simulink model "Bulker4_Main"  (R2023b)
settings: Solver=ode4  StartTime=0.0  StopTime=3600  FixedStep=0.01  RelTol=1e-3
StopFcn:
  | post_plot_bulker
undefined symbols (not defined in the file or in its folder): I, LOS, PD, S, x0, x_Curve, y_Curve
libraries: simulink x6, simulink_extras x1, mpclib x1
settings Model: SimulationMode=accelerator  Creator=HP  LastModifiedBy=myozi
settings SolverCC: AlgebraicLoopSolver=TrustRegion
settings DebuggingCC: UnconnectedInputMsg=warning  UnconnectedOutputMsg=warning  UnconnectedLineMsg=warning
settings ModelReferenceCC: EnableRefExpFcnMdlSchedulingChecks=on

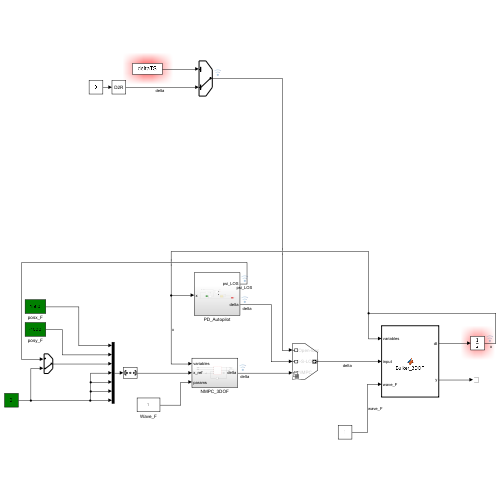
[thumbnail: Simulink's stored preview of the top-level diagram]
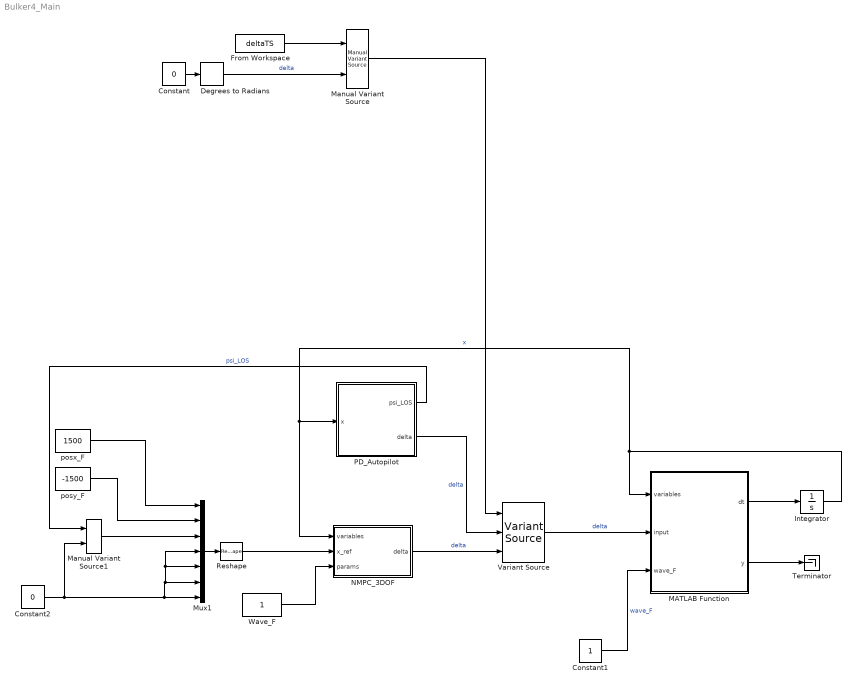
== system Bulker4_Main ==
  Constant : Constant  Value=0
  Constant1 : Constant
  Constant2 : Constant  Value=0
  Degrees to Radians : simulink_extras/Transformations/Degrees to Radians
  From Workspace : FromWorkspace  VariableName=deltaTS  OutputAfterFinalValue=Holding final value
  Integrator : Integrator  InitialCondition=x0
  MATLAB Function : MATLAB Function  TreatAsAtomicUnit=on
  Manual Variant Source : simulink/Signal Routing/Manual Variant Source  NumChoices=2  LabelModeActiveChoice=V_2
  Manual Variant Source1 : simulink/Signal Routing/Manual Variant Source  NumChoices=2  LabelModeActiveChoice=V_2
  Mux1 : Mux  Inputs=7
  NMPC_3DOF : Subsystem  VariantControl=Variant
  PD_Autopilot : Subsystem
  Reshape : Reshape  OutputDimensionality=Row vector (2-D)
  Terminator : Terminator
  Variant Source : VariantSource  VariantControlMode=label  LabelModeActiveChoice=I-S-LOS-PD  ShowConditionOnBlock=on
  Wave_F : Constant
  posx_F : Constant  Value=1500
  posy_F : Constant  Value=-1500
  wires:
  MATLAB Function/1(dt) -> Integrator/1
  Integrator/1 -> MATLAB Function/1(variables), PD_Autopilot/1(x), NMPC_3DOF/1(variables)  "x"
  Constant/1 -> Degrees to Radians/1
  Degrees to Radians/1 -> Manual Variant Source/2  "delta"
  Constant1/1 -> MATLAB Function/3(wave_F)  "wave_F"
  MATLAB Function/2(y) -> Terminator/1
  Variant Source/1 -> MATLAB Function/2(input)  "delta"
  Wave_F/1 -> NMPC_3DOF/3(params)
  Reshape/1 -> NMPC_3DOF/2(x_ref)
  NMPC_3DOF/1(delta) -> Variant Source/3  "delta"
  posy_F/1 -> Mux1/2
  Constant2/1 -> Manual Variant Source1/2, Mux1/6, Mux1/5, Mux1/4, Mux1/7
  Mux1/1 -> Reshape/1
  posx_F/1 -> Mux1/1
  PD_Autopilot/1(psi_LOS) -> Manual Variant Source1/1  "psi_LOS"
  PD_Autopilot/2(delta) -> Variant Source/2  "delta"
  Manual Variant Source1/1 -> Mux1/3
  Manual Variant Source/1 -> Variant Source/1
  From Workspace/1 -> Manual Variant Source/1

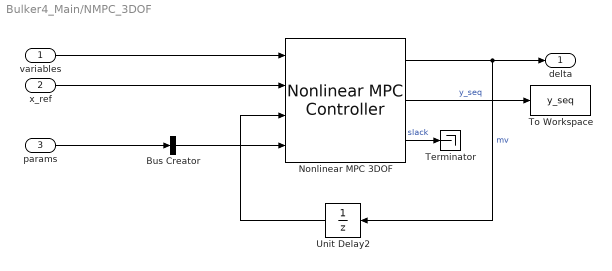
== system Bulker4_Main/NMPC_3DOF ==
  variables : Inport
  x_ref : Inport  Port=2
  params : Inport  Port=3
  Bus Creator : BusCreator  Inputs=1  OutDataTypeStr=Bus: params_bus_object  NonVirtualBus=on
      settings: InheritFromInputs=off
  Nonlinear MPC 3DOF : mpclib/Nonlinear MPC Controller  SCDEnableBlockLinearizationSpecification=on  nlmpcobj=bulker_nmpc_3_delta  UseObjectTs=off  TsControl=BlockTs  md_enabled=off  mvtarget_enabled=off  param_enabled=on  cost_enabled=off  mvseq_enabled=off  stateseq_enabled=off  ovseq_enabled=on  slack_enabled=on  status_enabled=off  ov_min=off  ov_max=off  mv_min=off  mv_max=off  mvrate_min=off  mvrate_max=off  state_min=off  state_max=off  ov_weight=off  mv_weight=off  mvrate_weight=off  ecr_weight=off  nlp_initialize=off
  Terminator : Terminator
  To Workspace : ToWorkspace  VariableName=y_seq  SaveFormat=Timeseries  SampleTime=-1
  Unit Delay2 : UnitDelay  SampleTime=-1  HasFrameUpgradeWarning=on
  delta : Outport  VectorParamsAs1DForOutWhenUnconnected=off
  wires:
  Nonlinear MPC 3DOF/1 -> Unit Delay2/1, delta/1  "mv"
  x_ref/1 -> Nonlinear MPC 3DOF/2
  variables/1 -> Nonlinear MPC 3DOF/1
  Unit Delay2/1 -> Nonlinear MPC 3DOF/3
  params/1 -> Bus Creator/1
  Bus Creator/1 -> Nonlinear MPC 3DOF/4
  Nonlinear MPC 3DOF/2 -> To Workspace/1  "y_seq"
  Nonlinear MPC 3DOF/3 -> Terminator/1  "slack"

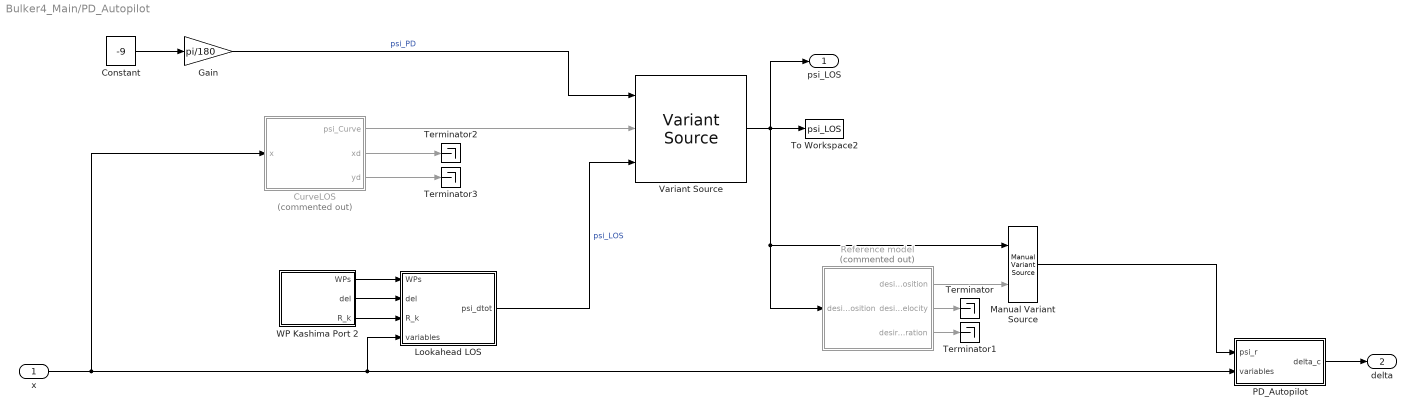
== system Bulker4_Main/PD_Autopilot ==
  x : Inport
  Constant : Constant  Value=-9
  CurveLOS : Subsystem  Commented=on
  Gain : Gain  Gain=pi/180
  Lookahead LOS : Subsystem
  Manual Variant Source : simulink/Signal Routing/Manual Variant Source  NumChoices=2  LabelModeActiveChoice=V_1
  PD_Autopilot : Subsystem  mask{K_P=3, T_D=100, T_E=1.74, delta_max=35, delta_rate=2.34}
      mask prompts: K_P "Proportional Gain :                               K_P"; T_D "Differential Time Constant : K_P*K_D = T_D"; T_E "Rudder Time Constant :                        T_E"; delta_max "Maximum Rudder Angle : delta_max (deg)"; delta_rate "Rudder Rate Limit : delta_rate (deg/s)"
      mask DialogControl Container3 Prompt: Rudder Limits
  Reference model : Subsystem  Commented=on  mask(3rd-order reference model){v_max=1.0, zeta_d=1.0, w_d=0.025}
      mask prompts: v_max "Max. velocity:"; zeta_d "Relative damping ratio:"; w_d "Natural frequency:"
      mask help: 3rd-order reference model with velocity saturation.
      mask Display:
      | disp('3rd order \nLP-filter')
      | port_label('output', 3, 'acc_d')
      | port_label('output', 2, 'vel_d')
      | port_label('output', 1, 'mag_d')
      | port_label('input', 1, 'ref')
  Terminator{,1..3} (4 alike) : Terminator
  To Workspace2 : ToWorkspace  VariableName=psi_LOS  SaveFormat=Timeseries  SampleTime=-1
  Variant Source : VariantSource  VariantControlMode=label  LabelModeActiveChoice=PD_Only  ShowConditionOnBlock=on
  WP Kashima Port 2 : Subsystem  mask{X_wp=[-200 1500 3000 110000 120000 300000], Y_wp=[30 -250 -1000 -70000 -90000 -300000], del=400, R_k_min=1.5*178, R_k_max=3*178}
      mask prompts: X_wp "X-Coordinates : X_wp [m]"; Y_wp "Y-Coordinates: Y_wp [m]"; del "Lookahead Distance : del (m)"; R_k_min "Radius of Circle of Acceptance : R_k Minimum (m)"; R_k_max "Radius of Circle of Acceptance : R_k Max (m)"
      mask DialogControl ParameterGroupVar Prompt: Waypoints
  psi_LOS : Outport  VectorParamsAs1DForOutWhenUnconnected=off
  delta : Outport  Port=2  VectorParamsAs1DForOutWhenUnconnected=off
  wires:
  WP Kashima Port 2/3(R_k) -> Lookahead LOS/3(R_k)
  WP Kashima Port 2/2(del) -> Lookahead LOS/2(del)
  PD_Autopilot/1(delta_c) -> delta/1
  WP Kashima Port 2/1(WPs) -> Lookahead LOS/1(WPs)
  x/1 -> CurveLOS/1(x), PD_Autopilot/2(variables), Lookahead LOS/4(variables)
  Constant/1 -> Gain/1
  Variant Source/1 -> Manual Variant Source/1, Reference model/1(desired position), psi_LOS/1, To Workspace2/1
  CurveLOS/1(psi_Curve) -> Variant Source/2
  CurveLOS/2(xd) -> Terminator2/1
  CurveLOS/3(yd) -> Terminator3/1
  Gain/1 -> Variant Source/1  "psi_PD"
  Lookahead LOS/1(psi_dtot) -> Variant Source/3  "psi_LOS"
  Reference model/1("desired position ") -> Manual Variant Source/2
  Reference model/2(desired velocity) -> Terminator/1
  Reference model/3(desired acceleration) -> Terminator1/1
  Manual Variant Source/1 -> PD_Autopilot/1(psi_r)

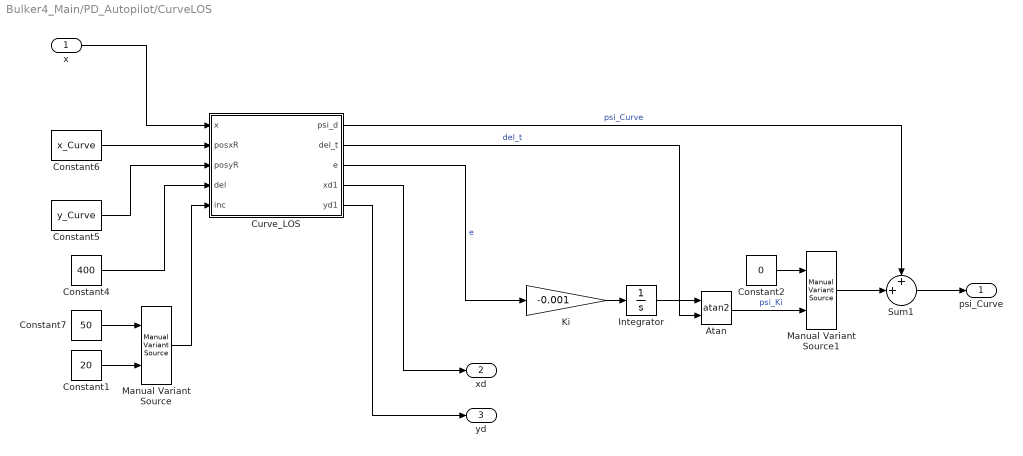
== system Bulker4_Main/PD_Autopilot/CurveLOS ==
  x : Inport
  Atan : Trigonometry  Operator=atan2
  Constant1 : Constant  Value=20
  Constant2 : Constant  Value=0
  Constant4 : Constant  Value=400
  Constant5 : Constant  Value=y_Curve
  Constant6 : Constant  Value=x_Curve
  Constant7 : Constant  Value=50
  Curve_LOS : MATLAB Function  TreatAsAtomicUnit=on
  Integrator : Integrator
  Ki : Gain  Gain=-0.001
  Manual Variant Source : simulink/Signal Routing/Manual Variant Source  NumChoices=2  LabelModeActiveChoice=V_2
  Manual Variant Source1 : simulink/Signal Routing/Manual Variant Source  NumChoices=2  LabelModeActiveChoice=V_2
  Sum1 : Sum  Inputs=++|
  psi_Curve : Outport  VectorParamsAs1DForOutWhenUnconnected=off
  xd : Outport  Port=2  VectorParamsAs1DForOutWhenUnconnected=off
  yd : Outport  Port=3  VectorParamsAs1DForOutWhenUnconnected=off
  wires:
  Constant5/1 -> Curve_LOS/3(posyR)
  Curve_LOS/2(del_t) -> Atan/2  "del_t"
  Constant7/1 -> Manual Variant Source/1
  Constant6/1 -> Curve_LOS/2(posxR)
  Curve_LOS/1(psi_d) -> Sum1/1  "psi_Curve"
  Constant4/1 -> Curve_LOS/4(del)
  Curve_LOS/3(e) -> Ki/1  "e"
  x/1 -> Curve_LOS/1(x)
  Integrator/1 -> Atan/1
  Ki/1 -> Integrator/1
  Constant2/1 -> Manual Variant Source1/1
  Atan/1 -> Manual Variant Source1/2  "psi_Ki"
  Manual Variant Source1/1 -> Sum1/2
  Sum1/1 -> psi_Curve/1
  Curve_LOS/4(xd1) -> xd/1
  Curve_LOS/5(yd1) -> yd/1
  Constant1/1 -> Manual Variant Source/2
  Manual Variant Source/1 -> Curve_LOS/5(inc)

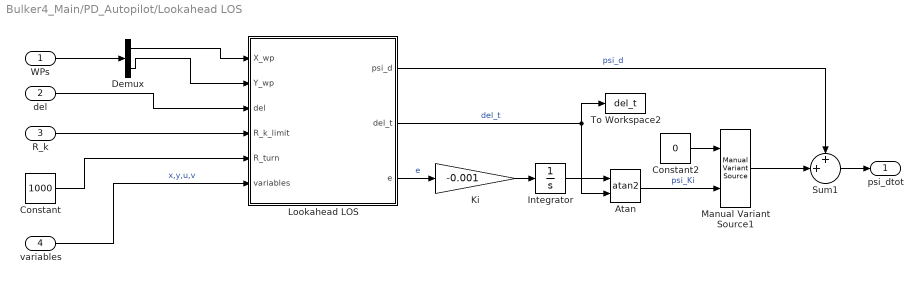
== system Bulker4_Main/PD_Autopilot/Lookahead LOS ==
  WPs : Inport
  del : Inport  Port=2
  R_k : Inport  Port=3
  variables : Inport  Port=4
  Atan : Trigonometry  Operator=atan2
  Constant : Constant  Value=1000
  Constant2 : Constant  Value=0
  Demux : Demux  Outputs=2
  Integrator : Integrator
  Ki : Gain  Gain=-0.001
  Lookahead LOS : Subsystem  Variant=on  VariantControlMode=label  VariantControl=Choice  LabelModeActiveChoice=varient3
  Manual Variant Source1 : simulink/Signal Routing/Manual Variant Source  NumChoices=2  LabelModeActiveChoice=V_2
  Sum1 : Sum  Inputs=++|
  To Workspace2 : ToWorkspace  VariableName=del_t  SaveFormat=Timeseries  SampleTime=-1
  psi_dtot : Outport  VectorParamsAs1DForOutWhenUnconnected=off
  wires:
  Lookahead LOS/1(psi_d) -> Sum1/1  "psi_d"
  R_k/1 -> Lookahead LOS/4(R_k_limit)
  variables/1 -> Lookahead LOS/6(variables)  "x,y,u,v"
  del/1 -> Lookahead LOS/3(del)
  WPs/1 -> Demux/1
  Demux/1 -> Lookahead LOS/1(X_wp)
  Demux/2 -> Lookahead LOS/2(Y_wp)
  Constant/1 -> Lookahead LOS/5(R_turn)
  Lookahead LOS/2(del_t) -> Atan/2, To Workspace2/1  "del_t"
  Lookahead LOS/3(e) -> Ki/1  "e"
  Sum1/1 -> psi_dtot/1
  Integrator/1 -> Atan/1
  Ki/1 -> Integrator/1
  Atan/1 -> Manual Variant Source1/2  "psi_Ki"
  Manual Variant Source1/1 -> Sum1/2
  Constant2/1 -> Manual Variant Source1/1

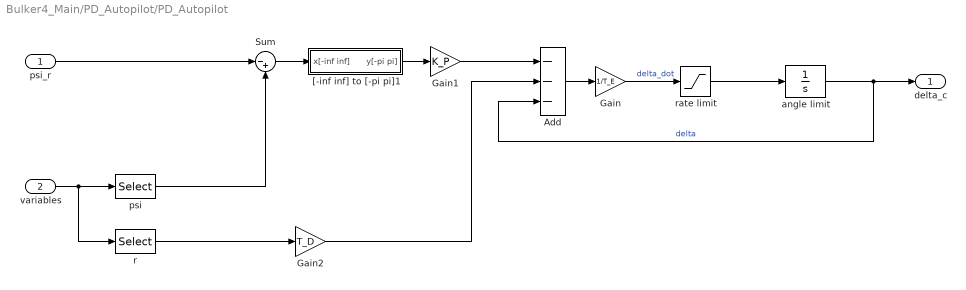
== system Bulker4_Main/PD_Autopilot/PD_Autopilot ==
  psi_r : Inport
  variables : Inport  Port=2
  Add : Sum  Inputs=---
  Gain : Gain  Gain=1/T_E
  Gain1 : Gain  Gain=K_P
  Gain2 : Gain  Gain=T_D
  Sum : Sum  Inputs=|-+
  "[-inf inf] to [-pi pi]1" : Subsystem
  angle limit : Integrator  LimitOutput=on  UpperSaturationLimit=delta_max*pi/180  LowerSaturationLimit=-delta_max*pi/180
  psi : Selector  InputPortWidth=7  IndexOptions=Index vector (dialog)  Indices=[3]  OutputSizes=1
  r : Selector  InputPortWidth=7  IndexOptions=Index vector (dialog)  Indices=[6]  OutputSizes=1
  rate limit : Saturate  UpperLimit=delta_rate*pi/180  LowerLimit=-delta_rate*pi/180
  delta_c : Outport  VectorParamsAs1DForOutWhenUnconnected=off
  wires:
  psi_r/1 -> Sum/1
  Add/1 -> Gain/1
  Gain1/1 -> Add/1
  Sum/1 -> "[-inf inf] to [-pi pi]1"/1(x[-inf inf])
  Gain/1 -> rate limit/1  "delta_dot"
  angle limit/1 -> Add/3, delta_c/1  "delta"
  Gain2/1 -> Add/2
  "[-inf inf] to [-pi pi]1"/1(y[-pi pi]) -> Gain1/1
  variables/1 -> r/1, psi/1
  rate limit/1 -> angle limit/1
  psi/1 -> Sum/2
  r/1 -> Gain2/1

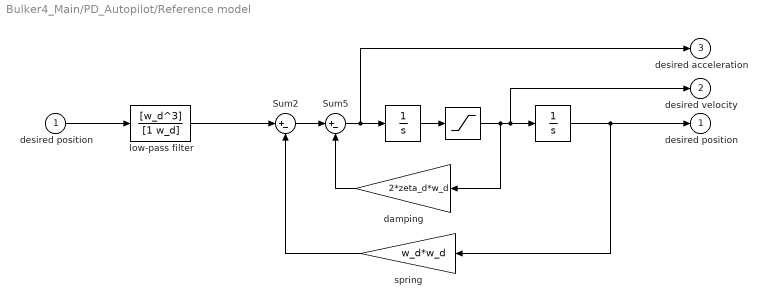
== system Bulker4_Main/PD_Autopilot/Reference model ==
  desired position : Inport
  "    " : TransferFcn  Denominator=[1 0]
  "       " : Saturate  UpperLimit=v_max  LowerLimit=-v_max
  "         " : TransferFcn  Denominator=[1 0]
  Sum2 : Sum  Inputs=|+-  InputSameDT=on  SaturateOnIntegerOverflow=on  OutDataTypeStr=Inherit: Same as first input
  Sum5 : Sum  Inputs=|+-  InputSameDT=on  SaturateOnIntegerOverflow=on  OutDataTypeStr=Inherit: Same as first input
  damping : Gain  Gain=2*zeta_d*w_d  SaturateOnIntegerOverflow=on  OutDataTypeStr=Inherit: Same as input  ParamDataTypeStr=Inherit: Same as input
  low-pass filter : TransferFcn  Numerator=[w_d^3]  Denominator=[1 w_d]
  spring : Gain  Gain=w_d*w_d  SaturateOnIntegerOverflow=on  OutDataTypeStr=Inherit: Same as input  ParamDataTypeStr=Inherit: Same as input
  "desired position " : Outport  InitialOutput=0  VectorParamsAs1DForOutWhenUnconnected=off
  desired velocity : Outport  Port=2  InitialOutput=0  VectorParamsAs1DForOutWhenUnconnected=off
  desired acceleration : Outport  Port=3  InitialOutput=0  VectorParamsAs1DForOutWhenUnconnected=off
  wires:
  "       "/1 -> desired velocity/1, "    "/1, damping/1
  Sum5/1 -> desired acceleration/1, "         "/1
  desired position/1 -> low-pass filter/1
  low-pass filter/1 -> Sum2/1
  Sum2/1 -> Sum5/1
  spring/1 -> Sum2/2
  "    "/1 -> spring/1, "desired position "/1
  "         "/1 -> "       "/1
  damping/1 -> Sum5/2

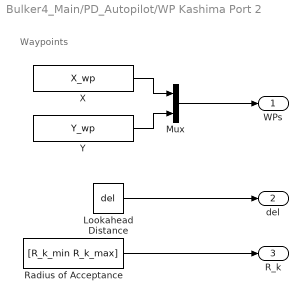
== system Bulker4_Main/PD_Autopilot/WP Kashima Port 2 ==
  note: Waypoints
  Lookahead Distance : Constant  Value=del
  Mux : Mux  Inputs=2
  Radius of Acceptance : Constant  Value=[R_k_min R_k_max]
  X : Constant  Value=X_wp
  Y : Constant  Value=Y_wp
  WPs : Outport  VectorParamsAs1DForOutWhenUnconnected=off
  del : Outport  Port=2  VectorParamsAs1DForOutWhenUnconnected=off
  R_k : Outport  Port=3  VectorParamsAs1DForOutWhenUnconnected=off
  wires:
  Y/1 -> Mux/2
  X/1 -> Mux/1
  Radius of Acceptance/1 -> R_k/1
  Lookahead Distance/1 -> del/1
  Mux/1 -> WPs/1

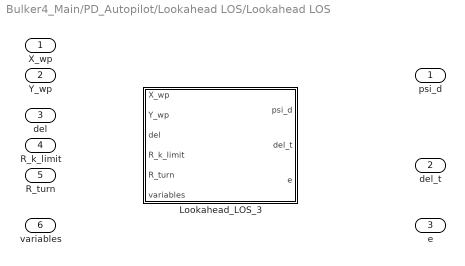
== system Bulker4_Main/PD_Autopilot/Lookahead LOS/Lookahead LOS ==
  X_wp : Inport
  Y_wp : Inport  Port=2
  del : Inport  Port=3
  R_k_limit : Inport  Port=4
  R_turn : Inport  Port=5
  variables : Inport  Port=6
  Lookahead_LOS_3 : MATLAB Function  TreatAsAtomicUnit=on  VariantControl=varient3
  psi_d : Outport  VectorParamsAs1DForOutWhenUnconnected=off
  del_t : Outport  Port=2  VectorParamsAs1DForOutWhenUnconnected=off
  e : Outport  Port=3  VectorParamsAs1DForOutWhenUnconnected=off

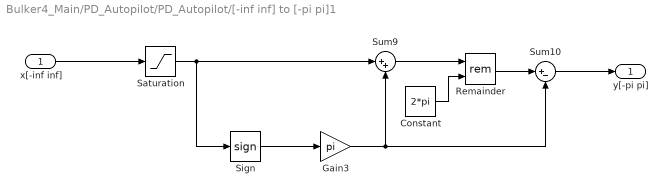
== system Bulker4_Main/PD_Autopilot/PD_Autopilot/[-inf inf] to [-pi pi]1 ==
  x[-inf inf] : Inport
  Constant : Constant  Value=2*pi
  Gain3 : Gain  Gain=pi
  Remainder : Math  Operator=rem  SignedPower=on
  Saturation : Saturate  UpperLimit=1e10  LowerLimit=-1e10
  Sign : Signum
  Sum10 : Sum  Inputs=|+-
  Sum9 : Sum  Inputs=|++
  y[-pi pi] : Outport  VectorParamsAs1DForOutWhenUnconnected=off
  wires:
  Sum9/1 -> Remainder/1
  x[-inf inf]/1 -> Saturation/1
  Remainder/1 -> Sum10/1
  Sum10/1 -> y[-pi pi]/1
  Sign/1 -> Gain3/1
  Saturation/1 -> Sum9/1, Sign/1
  Gain3/1 -> Sum9/2, Sum10/2
  Constant/1 -> Remainder/2

== matlab function Bulker4_Main/MATLAB Function ==
  data: dt output; variables input; y output; input input; wave_F input
function [dt, y] = Bulker_3DOF(variables,input,wave_F)
params = wave_F;
[dt, y] = Bulker2_StateFunction_3DOF_delta(variables,input,params);

== matlab function Bulker4_Main/PD_Autopilot/Lookahead LOS/Lookahead LOS/Lookahead_LOS_3 ==
  settings: updateMethod=DISCRETE
  data: X_wp input; Y_wp input; del input; R_k_limit input; R_turn input; psi_d output; variables input; del_t output; e output
function [psi_d, del_t, e]   = straightLOS_Sim(X_wp,Y_wp,del,R_k_limit,R_turn,variables)

[psi_d, del_t, e]   = straightLOS(X_wp,Y_wp,del,R_k_limit,R_turn,variables);

== matlab function Bulker4_Main/PD_Autopilot/CurveLOS/Curve_LOS ==
  data: x input; psi_d output; posxR input; posyR input; del input; inc input; del_t output; e output; xd1 output; yd1 output
function [psi_d, del_t, e, xd1, yd1] = curveLOS_sim(x, posxR, posyR, del, inc)
% inc >> increased step >> should be represent the Total Prediction Horizon Time
[psi_d, xd, yd,del_t,e] = curveLOS(x, posxR, posyR, del, inc);
xd1 = xd(2);
yd1 = yd(2);
